simulink model "P2PHVDCMMC"  (R2024a)
settings: Solver=FixedStepDiscrete  StartTime=0.0  StopTime=10  RelTol=1e-3
PreLoadFcn:
  | % HVDCMMCInterconnectionParam
StartFcn:
  | tic
StopFcn:
  | toc
values from neighbouring files (symbols this model uses):
  C_PM = 1.758e-3    (= 0.001758)    [P2PHVDCMMCcode.m]    (also in SFu.mat)
  Cg = 50e-9    (= 5e-08)    [P2PHVDCMMCcode.m]    (also in SFu.mat)
  Fc = Fnom*3.37    (= 168.5)    [P2PHVDCMMCcode.m]    (also in SFu.mat)
  Fnom = 50    [P2PHVDCMMCcode.m]    (also in SFu.mat)
  HRM = 1    [SFu.mat]
  Ki_Ireg = 6    [P2PHVDCMMCcode.m]    (also in SFu.mat)
  Ki_Preg = 1.0    (= 1)    [P2PHVDCMMCcode.m]    (also in SFu.mat)
  Ki_Qreg = 1.0    (= 1)    [P2PHVDCMMCcode.m]    (also in SFu.mat)
  Ki_VDCreg = 100    [P2PHVDCMMCcode.m]    (also in SFu.mat)
  Kp_Ireg = 0.6    [P2PHVDCMMCcode.m]    (also in SFu.mat)
  Kp_Preg = 0.5/3    (= 0.166666666667)    [P2PHVDCMMCcode.m]    (also in SFu.mat)
  Kp_Qreg = 0.5/3    (= 0.166666666667)    [P2PHVDCMMCcode.m]    (also in SFu.mat)
  Kp_VDCreg = 4    [P2PHVDCMMCcode.m]    (also in SFu.mat)
  L_cable = 15e-3    (= 0.015)    [P2PHVDCMMCcode.m]    (also in SFu.mat)
  Larm = Larm_pu*(Zb_ac/(2*pi*Fnom))    [P2PHVDCMMCcode.m]    (also in SFu.mat = 0.0529455974536)
  Larm_pu = 0.15    [P2PHVDCMMCcode.m]    (also in SFu.mat)
  Lff = Larm_pu/2    (= 0.075)    [P2PHVDCMMCcode.m]    (also in SFu.mat)
  Limits_Ireg = [ 2.0  -2.0]    [P2PHVDCMMCcode.m]    (also in SFu.mat = [2 -2])
  Limits_Preg = [ 1.2, 0.8 ]    [P2PHVDCMMCcode.m]    (also in SFu.mat = [1.2 0.8])
  Limits_Qreg = [ 0.25, -0.25 ]    [P2PHVDCMMCcode.m]    (also in SFu.mat = [0.25 -0.25])
  Limits_VDCreg = [ 2.0  -2.0]    [P2PHVDCMMCcode.m]    (also in SFu.mat = [2 -2])
  Lxfo = 0.12    [P2PHVDCMMCcode.m]    (also in SFu.mat)
  N = 1    [P2PHVDCMMCcode.m]    (also in SFu.mat)
  Nb_PM = 36    [P2PHVDCMMCcode.m]    (also in SFu.mat)
  Pnom = 1000e6    (= 1000000000)    [P2PHVDCMMCcode.m]    (also in SFu.mat)
  R_cable = 0.5    [P2PHVDCMMCcode.m]    (also in SFu.mat)
  R_startup = 400    [P2PHVDCMMCcode.m]    (also in SFu.mat)
  Rarm = Rarm_pu*Zb_ac    [P2PHVDCMMCcode.m]    (also in SFu.mat = 0.1663335)
  Rff = Rarm_pu/2    (= 0.00075)    [P2PHVDCMMCcode.m]    (also in SFu.mat)
  Rg = 100    [P2PHVDCMMCcode.m]    (also in SFu.mat)
  Rxfo = 0.003    [P2PHVDCMMCcode.m]    (also in SFu.mat)
  S =     [SFu.mat]
  Slope_Qref = 0.5    [P2PHVDCMMCcode.m]    (also in SFu.mat)
  Slope_Vdc_ref = Vnom_dc/5    (= 128000)    [P2PHVDCMMCcode.m]    (also in SFu.mat)
  Tfault = 9999    [SFu.mat]
  Ts = Ts_Control    (= 4e-05)    [P2PHVDCMMCcode.m]    (also in SFu.mat)
  Ts_Control = 40e-6    (= 4e-05)    [P2PHVDCMMCcode.m]    (also in SFu.mat)
  Ts_dqn = 2e-5    (= 2e-05)    [P2PHVDCMMCcode.m]    (also in SFu.mat)
  Ts_Power = 20e-6    (= 2e-05)    [P2PHVDCMMCcode.m]    (also in SFu.mat)
  Vnom_dc = 640e3    (= 640000)    [P2PHVDCMMCcode.m]    (also in SFu.mat)
  Vnom_prim = 400e3    (= 400000)    [P2PHVDCMMCcode.m]    (also in SFu.mat)
  Vnom_sec = 333e3    (= 333000)    [P2PHVDCMMCcode.m]    (also in SFu.mat)
  Ws = 314.159265359    [SFu.mat]
undefined symbols (not defined in the file or in its folder): DiscIntNeverNeededParam, Discrete, DQN_Lib, gcbh, Int_DQNc_Mat, Mult_DQNc_Mat, Pcc, sps, sps_rtmsupport, spsMeanValueVariableFrequencyModel, spsPLL3phModel, SY3
libraries: simulink x38, spsControlledVoltageSourceLib x30, spsVoltageMeasurementLib x21, spsIdealSwitchLib x21, powerlib_extras x12, spsSecondOrderFilterLib x12, spsCurrentMeasurementLib x12, spsdq0toabcLib x9, spsMeanLib x8, spsMeanVariableFrequencyLib x8, spsabctodq0Lib x8, spsThreePhaseSeriesRLCBranchLib x7
(part 12 of 13)

== matlab function P2PHVDCMMC/Subsystem4/ACinv/Mult_DQNc_Mat3 ==
  data: Xdcpnz_c input; Ydcpnz_c input; N parameter; HrmDbl parameter; Zdcpnz_c output
function Zdcpnz_c    = fMultDQNc(Xdcpnz_c, Ydcpnz_c, N, HrmDbl)
    Zdcpnz_c = complex(zeros(3,2*N+1));

    persistent T132;
    persistent T213;
    persistent T231;
    persistent T321;
    persistent T312;
    persistent Sas;
    persistent Ssa;

    if(isempty(T132)) 
        T132 = [1 0 0; 0 0 1; 0 1 0];
        T213 = [0 1 0; 1 0 0; 0 0 1];
        T231 = [0 1 0; 0 0 1; 1 0 0];
        T321 = [0 0 1; 0 1 0; 1 0 0];
        T312 = [0 0 1; 1 0 0; 0 1 0];

        a = -0.5+0.866i;
        a2 = -0.5-0.866i;
        Sas = [1,a,a2;1,a2,a;1,1,1]/3;
        Ssa = eye(3)/(Sas);
    end

%%%%%%%%%%%%%%%%%%%%%%%%%%%%%%

    Zdcpnz_c(:,1) = Sas*(Ssa*Xdcpnz_c(:,1).*Ssa*Ydcpnz_c(:,1));

    sX = size(Xdcpnz_c,2);
    Xdcpnz_c = [Xdcpnz_c zeros(3,N+1-sX)];

    sY = size(Ydcpnz_c,2);
    Ydcpnz_c = [Ydcpnz_c zeros(3,N+1-sY)];

       
    for h = 1 : 2*N
        if(h<=N)

            Zdcpnz_c(3,1) = Zdcpnz_c(3,1) + 0.5*real(Xdcpnz_c(:,h+1)'*Ydcpnz_c(:,h+1));


            Zdcpnz_c(3,2*h+1) = Zdcpnz_c(3,2*h+1) + 0.5*Xdcpnz_c(1,h+1)*Ydcpnz_c(2,h+1)*exp(-1i*pi/2);

            Zdcpnz_c(1:2,1) = Zdcpnz_c(1:2,1) + 0.25*abs(Xdcpnz_c(1,h+1))*abs(Ydcpnz_c(2,h+1))*[1;1].*exp(1i*((-angle(Xdcpnz_c(1,h+1))+angle(Ydcpnz_c(2,h+1)))*[1;-1]));
            Zdcpnz_c(1:2,1) = Zdcpnz_c(1:2,1) + 0.25*abs(Xdcpnz_c(1,h+1))*abs(Ydcpnz_c(3,h+1))*[1;1].*exp(1i*((-angle(Xdcpnz_c(1,h+1))+angle(Ydcpnz_c(3,h+1)))*[-1;1]));


            Zdcpnz_c(3,2*h+1) = Zdcpnz_c(3,2*h+1) + 0.5*Xdcpnz_c(2,h+1)*Ydcpnz_c(1,h+1)*exp(-1i*pi/2);


            Zdcpnz_c(1:2,1) = Zdcpnz_c(1:2,1) + 0.25*abs(Xdcpnz_c(2,h+1))*abs(Ydcpnz_c(1,h+1))*[1;1].*exp(1i*((-angle(Xdcpnz_c(2,h+1))+angle(Ydcpnz_c(1,h+1)))*[-1;1]));
            Zdcpnz_c(1:2,1) = Zdcpnz_c(1:2,1) + 0.25*abs(Xdcpnz_c(2,h+1))*abs(Ydcpnz_c(3,h+1))*[1;1].*exp(1i*((-angle(Xdcpnz_c(2,h+1))+angle(Ydcpnz_c(3,h+1)))*[1;-1]));
            
            Zdcpnz_c(1:2,1) = Zdcpnz_c(1:2,1) + 0.25*abs(Xdcpnz_c(3,h+1))*abs(Ydcpnz_c(1,h+1))*[1;1].*exp(1i*((-angle(Xdcpnz_c(3,h+1))+angle(Ydcpnz_c(1,h+1)))*[1;-1]));
            Zdcpnz_c(1:2,1) = Zdcpnz_c(1:2,1) + 0.25*abs(Xdcpnz_c(3,h+1))*abs(Ydcpnz_c(2,h+1))*[1;1].*exp(1i*((-angle(Xdcpnz_c(3,h+1))+angle(Ydcpnz_c(2,h+1)))*[-1;+1]));

            %%%%%%%%%%%%%%%%% POSITIVE (Ydc*Xp) %%%%%%%%%%%%%%%%%%%
            Zdcpnz_c(:,h+1) = Zdcpnz_c(:,h+1) + T312*Ydcpnz_c(:,1)*Xdcpnz_c(1,h+1); %[0 0 1; 1 0 0; 0 1 0]
            %%%%%%%%%%%%%%%%% POSITIVE (Xdc*Yp) %%%%%%%%%%%%%%%%%%%
            Zdcpnz_c(:,h+1) = Zdcpnz_c(:,h+1) + T312*Xdcpnz_c(:,1)*Ydcpnz_c(1,h+1);
            %%%%%%%%%%%%%%%%% NEGATIVE (Ydc*Xn) %%%%%%%%%%%%%%%%%%%
            Zdcpnz_c(:,h+1) = Zdcpnz_c(:,h+1) + T231*Ydcpnz_c(:,1)*Xdcpnz_c(2,h+1);
            %%%%%%%%%%%%%%%%% NEGATIVE (Xdc*Yn) %%%%%%%%%%%%%%%%%%%
            Zdcpnz_c(:,h+1) = Zdcpnz_c(:,h+1) + T231*Xdcpnz_c(:,1)*Ydcpnz_c(2,h+1);
            %%%%%%%%%%%%%%%%%%%%%%%%%%%%%%%%%%%%%%%%%%%%%%%%%%%%%%
            Zdcpnz_c(:,h+1) = Zdcpnz_c(:,h+1) + Ydcpnz_c(:,1)*Xdcpnz_c(3,h+1);
            %%%%%%%%%%%%%%%%%%%%%%%%%%%%%%%%%%%%%%%%%%%%%%%%%%%%%%
            Zdcpnz_c(:,h+1) = Zdcpnz_c(:,h+1) + Xdcpnz_c(:,1)*Ydcpnz_c(3,h+1);
            
%%%%%%%%%%%%%%%%%%%%%% h<=N ODD %%%%%%%%%%%%%%%%%%%%%%%%%%%%%%%%%%%%%%%%%
            if(mod(h,2)==1) 
                %%%%%%%%%%%%%%%%% D3p (3ph+) %%%%%%%%%%%%%%%%%%%%%%%

                %&%%%%%%%%%%%%%%%%%%%%%%%%%% PP + NN %%%%%%%%%%%%%%%%%%%%%%%%%%%
                for i = 1 : h - 1
                   Zdcpnz_c(1,h+1) = Zdcpnz_c(1,h+1) +    0.5*( real(Xdcpnz_c(2,i+1))*imag(Ydcpnz_c(2,h-i+1)) + imag(Xdcpnz_c(2,i+1))*real(Ydcpnz_c(2,h-i+1)) );
                   Zdcpnz_c(1,h+1) = Zdcpnz_c(1,h+1) + 1i*0.5*( -real(Xdcpnz_c(2,i+1))*real(Ydcpnz_c(2,h-i+1)) + imag(Xdcpnz_c(2,i+1))*imag(Ydcpnz_c(2,h-i+1)) );

                   Zdcpnz_c(2,h+1) = Zdcpnz_c(2,h+1) +    0.5*( real(Xdcpnz_c(1,i+1))*imag(Ydcpnz_c(1,h-i+1)) + imag(Xdcpnz_c(1,i+1))*real(Ydcpnz_c(1,h-i+1)) );
                   Zdcpnz_c(2,h+1) = Zdcpnz_c(2,h+1) + 1i*0.5*( -real(Xdcpnz_c(1,i+1))*real(Ydcpnz_c(1,h-i+1)) + imag(Xdcpnz_c(1,i+1))*imag(Ydcpnz_c(1,h-i+1)) );
                end

                for i = 1 : N - h

                    Zdcpnz_c(3,h+1) = Zdcpnz_c(3,h+1) -    imag(0.5*Xdcpnz_c(1:2,i+1)'*Ydcpnz_c(1:2,i+h+1)) -    imag(0.5*Ydcpnz_c(1:2,i+1)'*Xdcpnz_c(1:2,i+h+1));
                    Zdcpnz_c(3,h+1) = Zdcpnz_c(3,h+1) + 1i*real(0.5*Xdcpnz_c(1:2,i+1)'*Ydcpnz_c(1:2,i+h+1)) + 1i*real(0.5*Ydcpnz_c(1:2,i+1)'*Xdcpnz_c(1:2,i+h+1));

                end
                %&%%%%%%%%%%%%%%%%%%%%%%%%%% PP + NN %%%%%%%%%%%%%%%%%%%%%%%%%%%

                for k = 1 : (N + mod(N+1,2) - h)/2
                    i = 2*k-1;
                    j = i+h;

                    Zdcpnz_c(1,h+1) = Zdcpnz_c(1,h+1) + (0.5*(Xdcpnz_c(:,i+1)'*T132*T213*Ydcpnz_c(:,j+1))*exp(+1i*pi/2)) ...
                                                      + (0.5*(Xdcpnz_c(:,j+1)'*T213*T132*Ydcpnz_c(:,i+1))*exp(-1i*pi/2))';

                    Zdcpnz_c(2,h+1) = Zdcpnz_c(2,h+1) + (0.5*(Xdcpnz_c(:,i+1)'*T132*T321*Ydcpnz_c(:,j+1))*exp(+1i*pi/2)) ...
                                                      + (0.5*(Xdcpnz_c(:,j+1)'*T321*T132*Ydcpnz_c(:,i+1))*exp(-1i*pi/2))';

                    Zdcpnz_c(3,h+1) = Zdcpnz_c(3,h+1) + (0.5*Xdcpnz_c(3,i+1)'*Ydcpnz_c(3,j+1)*exp(1i*pi/2)) ...
                                                      - (0.5*Xdcpnz_c(3,j+1)'*Ydcpnz_c(3,i+1)*exp(1i*pi/2))';
                end

                for k = 1 : (N + mod(N,2) - h - 1)/2
                    i = 2*k;
                    j = i+h;
                    
                    Zdcpnz_c(1,h+1) = Zdcpnz_c(1,h+1) + (0.5*(Xdcpnz_c(:,i+1)'*T132*T213*Ydcpnz_c(:,j+1))*exp(+1i*pi/2)) ...
                                                      + (0.5*(Xdcpnz_c(:,j+1)'*T213*T132*Ydcpnz_c(:,i+1))*exp(-1i*pi/2))';

                    Zdcpnz_c(2,h+1) = Zdcpnz_c(2,h+1) + (0.5*(Xdcpnz_c(:,i+1)'*T132*T321*Ydcpnz_c(:,j+1))*exp(+1i*pi/2)) ...
                                                      + (0.5*(Xdcpnz_c(:,j+1)'*T321*T132*Ydcpnz_c(:,i+1))*exp(-1i*pi/2))';

                    Zdcpnz_c(3,h+1) = Zdcpnz_c(3,h+1) + (0.5*Xdcpnz_c(3,i+1)'*Ydcpnz_c(3,j+1)*exp(1i*pi/2)) ...
                                                      - (0.5*Xdcpnz_c(3,j+1)'*Ydcpnz_c(3,i+1)*exp(1i*pi/2))';
                end

                for k = (h-1)/2:-1:1
                    i = k;
                    j = h-i;  

                    Zdcpnz_c(3,h+1) = Zdcpnz_c(3,h+1) + 0.5*(real(Xdcpnz_c(:,i+1))'*T213*imag(Ydcpnz_c(:,j+1)) + imag(Xdcpnz_c(:,i+1))'*T213*real(Ydcpnz_c(:,j+1)) ...
                                                           + real(Xdcpnz_c(:,j+1))'*T213*imag(Ydcpnz_c(:,i+1)) + imag(Xdcpnz_c(:,j+1))'*T213*real(Ydcpnz_c(:,i+1)));
                                                                                       
                    Zdcpnz_c(3,h+1) = Zdcpnz_c(3,h+1) + 1i*0.5*(-real(Xdcpnz_c(:,i+1))'*T213*real(Ydcpnz_c(:,j+1)) + imag(Xdcpnz_c(:,i+1))'*T213*imag(Ydcpnz_c(:,j+1)) ...
                                                           - real(Xdcpnz_c(:,j+1))'*T213*real(Ydcpnz_c(:,i+1)) + imag(Xdcpnz_c(:,j+1))'*T213*imag(Ydcpnz_c(:,i+1)));

                    Zdcpnz_c(1,h+1) = Zdcpnz_c(1,h+1) + 0.5*(real(Xdcpnz_c([1,3],i+1))'*[0 1; 1 0]*imag(Ydcpnz_c([1,3],j+1)) + imag(Xdcpnz_c([1,3],i+1))'*[0 1; 1 0]*real(Ydcpnz_c([1,3],j+1)) ...
                                                           + real(Xdcpnz_c([1,3],j+1))'*[0 1; 1 0]*imag(Ydcpnz_c([1,3],i+1)) + imag(Xdcpnz_c([1,3],j+1))'*[0 1; 1 0]*real(Ydcpnz_c([1,3],i+1)) );

                    Zdcpnz_c(1,h+1) = Zdcpnz_c(1,h+1) + 1i*0.5*(-real(Xdcpnz_c([1,3],i+1))'*[0 1; 1 0]*real(Ydcpnz_c([1,3],j+1)) + imag(Xdcpnz_c([1,3],i+1))'*[0 1; 1 0]*imag(Ydcpnz_c([1,3],j+1)) ...
                                                              - real(Xdcpnz_c([1,3],j+1))'*[0 1; 1 0]*real(Ydcpnz_c([1,3],i+1)) + imag(Xdcpnz_c([1,3],j+1))'*[0 1; 1 0]*imag(Ydcpnz_c([1,3],i+1)) );

                    Zdcpnz_c(2,h+1) = Zdcpnz_c(2,h+1) + 0.5*(real(Xdcpnz_c([2,3],i+1))'*[0 1; 1 0]*imag(Ydcpnz_c([2,3],j+1)) + imag(Xdcpnz_c([2,3],i+1))'*[0 1; 1 0]*real(Ydcpnz_c([2,3],j+1)) ...
                                                           + real(Xdcpnz_c([2,3],j+1))'*[0 1; 1 0]*imag(Ydcpnz_c([2,3],i+1)) + imag(Xdcpnz_c([2,3],j+1))'*[0 1; 1 0]*real(Ydcpnz_c([2,3],i+1)) );

                    Zdcpnz_c(2,h+1) = Zdcpnz_c(2,h+1) + 1i*0.5*(-real(Xdcpnz_c([2,3],i+1))'*[0 1; 1 0]*real(Ydcpnz_c([2,3],j+1)) + imag(Xdcpnz_c([2,3],i+1))'*[0 1; 1 0]*imag(Ydcpnz_c([2,3],j+1)) ...
                                                              - real(Xdcpnz_c([2,3],j+1))'*[0 1; 1 0]*real(Ydcpnz_c([2,3],i+1)) + imag(Xdcpnz_c([2,3],j+1))'*[0 1; 1 0]*imag(Ydcpnz_c([2,3],i+1)) );

                end
%%%%%%%%%%%%%%%%%%%%%% h<=N EVEN %%%%%%%%%%%%%%%%%%%%%%%%%%%%%%%%%%%%%%%%%           
            else  

                Zdcpnz_c(3,h+1) = Zdcpnz_c(3,h+1) + 0.5*imag(Xdcpnz_c(3,h/2+1)*Ydcpnz_c(3,h/2+1))           -0.5*1i*real(Xdcpnz_c(3,h/2+1)*Ydcpnz_c(3,h/2+1));
                Zdcpnz_c(1,h+1) = Zdcpnz_c(1,h+1) + 0.5*real(Xdcpnz_c(:,h/2+1))'*T321*imag(Ydcpnz_c(:,h/2+1)) + 0.5*imag(Xdcpnz_c(:,h/2+1))'*T321*real(Ydcpnz_c(:,h/2+1));
                Zdcpnz_c(1,h+1) = Zdcpnz_c(1,h+1) - 0.5*1i*real(Xdcpnz_c(:,h/2+1))'*T321*real(Ydcpnz_c(:,h/2+1)) + 0.5*1i*imag(Xdcpnz_c(:,h/2+1))'*T321*imag(Ydcpnz_c(:,h/2+1));
                Zdcpnz_c(2,h+1) = Zdcpnz_c(2,h+1) + 0.5*real(Xdcpnz_c(:,h/2+1))'*T132*imag(Ydcpnz_c(:,h/2+1)) + 0.5*imag(Xdcpnz_c(:,h/2+1))'*T132*real(Ydcpnz_c(:,h/2+1));
                Zdcpnz_c(2,h+1) = Zdcpnz_c(2,h+1) - 0.5*1i*real(Xdcpnz_c(:,h/2+1))'*T132*real(Ydcpnz_c(:,h/2+1)) + 0.5*1i*imag(Xdcpnz_c(:,h/2+1))'*T132*imag(Ydcpnz_c(:,h/2+1));
                
                for k = 1:N-h
                    i = k;
                    j = h+i;

                    Zdcpnz_c(1,h+1) = Zdcpnz_c(1,h+1) + 0.5*( - real(Xdcpnz_c(:,i+1))'*T231*imag(Ydcpnz_c(:,j+1)) + imag(Xdcpnz_c(:,i+1))'*T231*real(Ydcpnz_c(:,j+1)) ...
                                                              + real(Xdcpnz_c(:,j+1))'*T312*imag(Ydcpnz_c(:,i+1)) - imag(Xdcpnz_c(:,j+1))'*T312*real(Ydcpnz_c(:,i+1)));

                    Zdcpnz_c(1,h+1) = Zdcpnz_c(1,h+1) + 0.5*1i*( + real(Xdcpnz_c(:,i+1))'*T231*real(Ydcpnz_c(:,j+1)) + imag(Xdcpnz_c(:,i+1))'*T231*imag(Ydcpnz_c(:,j+1)) ...
                                                                 + real(Xdcpnz_c(:,j+1))'*T312*real(Ydcpnz_c(:,i+1)) + imag(Xdcpnz_c(:,j+1))'*T312*imag(Ydcpnz_c(:,i+1)));

                    Zdcpnz_c(2,h+1) = Zdcpnz_c(2,h+1) + 0.5*( - real(Xdcpnz_c(:,i+1))'*T312*imag(Ydcpnz_c(:,j+1)) + imag(Xdcpnz_c(:,i+1))'*T312*real(Ydcpnz_c(:,j+1)) ...
                                                              + real(Xdcpnz_c(:,j+1))'*T231*imag(Ydcpnz_c(:,i+1)) - imag(Xdcpnz_c(:,j+1))'*T231*real(Ydcpnz_c(:,i+1)));

                    Zdcpnz_c(2,h+1) = Zdcpnz_c(2,h+1) + 1i*0.5*( + real(Xdcpnz_c(:,i+1))'*T312*real(Ydcpnz_c(:,j+1)) + imag(Xdcpnz_c(:,i+1))'*T312*imag(Ydcpnz_c(:,j+1)) ...
                                                              + real(Xdcpnz_c(:,j+1))'*T231*real(Ydcpnz_c(:,i+1)) + imag(Xdcpnz_c(:,j+1))'*T231*imag(Ydcpnz_c(:,i+1)));

                    Zdcpnz_c(3,h+1) = Zdcpnz_c(3,h+1) + 0.5*(-real(Xdcpnz_c(:,i+1))'*imag(Ydcpnz_c(:,j+1))+imag(Xdcpnz_c(:,i+1))'*real(Ydcpnz_c(:,j+1)) ...
                                                             +real(Xdcpnz_c(:,j+1))'*imag(Ydcpnz_c(:,i+1))-imag(Xdcpnz_c(:,j+1))'*real(Ydcpnz_c(:,i+1)));

                    Zdcpnz_c(3,h+1) = Zdcpnz_c(3,h+1) + 0.5*1i*(+real(Xdcpnz_c(:,i+1))'*real(Ydcpnz_c(:,j+1))+imag(Xdcpnz_c(:,i+1))'*imag(Ydcpnz_c(:,j+1)) ...
                                                             +real(Xdcpnz_c(:,j+1))'*real(Ydcpnz_c(:,i+1))+imag(Xdcpnz_c(:,j+1))'*imag(Ydcpnz_c(:,i+1)));

                end

                for k = h/2-1:-1:1
                    i = k;
                    j = h-i;   

                    Zdcpnz_c(3,h+1) = Zdcpnz_c(3,h+1) +    0.5*(+real(Xdcpnz_c(:,i+1))'*T213*imag(Ydcpnz_c(:,j+1)) + real(Xdcpnz_c(:,j+1))'*T213*imag(Ydcpnz_c(:,i+1)) + imag(Xdcpnz_c(:,i+1))'*T213*real(Ydcpnz_c(:,j+1)) + imag(Xdcpnz_c(:,j+1))'*T213*real(Ydcpnz_c(:,i+1)));

                    Zdcpnz_c(3,h+1) = Zdcpnz_c(3,h+1) + 1i*0.5*(-real(Xdcpnz_c(:,i+1))'*T213*real(Ydcpnz_c(:,j+1)) - real(Xdcpnz_c(:,j+1))'*T213*real(Ydcpnz_c(:,i+1)) + imag(Xdcpnz_c(:,i+1))'*T213*imag(Ydcpnz_c(:,j+1)) + imag(Xdcpnz_c(:,j+1))'*T213*imag(Ydcpnz_c(:,i+1)));

                    Zdcpnz_c(1,h+1) = Zdcpnz_c(1,h+1) + 0.5*( + real(Xdcpnz_c(:,i+1))'*T321*imag(Ydcpnz_c(:,j+1)) + imag(Xdcpnz_c(:,i+1))'*T321*real(Ydcpnz_c(:,j+1)) ...
                                                              + real(Xdcpnz_c(:,j+1))'*T321*imag(Ydcpnz_c(:,i+1)) + imag(Xdcpnz_c(:,j+1))'*T321*real(Ydcpnz_c(:,i+1)));


                    Zdcpnz_c(1,h+1) = Zdcpnz_c(1,h+1) + 0.5*1i*( - real(Xdcpnz_c(:,i+1))'*T321*real(Ydcpnz_c(:,j+1)) + imag(Xdcpnz_c(:,i+1))'*T321*imag(Ydcpnz_c(:,j+1)) ...
                                                                 - real(Xdcpnz_c(:,j+1))'*T321*real(Ydcpnz_c(:,i+1)) + imag(Xdcpnz_c(:,j+1))'*T321*imag(Ydcpnz_c(:,i+1)));
                    
                    Zdcpnz_c(2,h+1) = Zdcpnz_c(2,h+1) + 0.5*( + real(Xdcpnz_c(:,i+1))'*T132*imag(Ydcpnz_c(:,j+1)) + imag(Xdcpnz_c(:,i+1))'*T132*real(Ydcpnz_c(:,j+1)) ...
                                                              + real(Xdcpnz_c(:,j+1))'*T132*imag(Ydcpnz_c(:,i+1)) + imag(Xdcpnz_c(:,j+1))'*T132*real(Ydcpnz_c(:,i+1)));

                    Zdcpnz_c(2,h+1) = Zdcpnz_c(2,h+1) + 1i*0.5*( - real(Xdcpnz_c(:,i+1))'*T132*real(Ydcpnz_c(:,j+1)) + imag(Xdcpnz_c(:,i+1))'*T132*imag(Ydcpnz_c(:,j+1)) ...
                                                                 - real(Xdcpnz_c(:,j+1))'*T132*real(Ydcpnz_c(:,i+1)) + imag(Xdcpnz_c(:,j+1))'*T132*imag(Ydcpnz_c(:,i+1)));

                end
            end
%%%%%%%%%%%%%%%%%%%%%%%%%%%% h>N  %%%%%%%%%%%%%%%%%%%%%%%%%%%%%%%%%%%%%%%%% 
        else %h>N
            if(HrmDbl)
            
                %%%%%%%%%%%%%%%%%%%%%%%%%%% PP + NN %%%%%%%%%%%%%%%%%%%%%%%%%%%
                for i = h-N : N
                    Zdcpnz_c(1,h+1) = Zdcpnz_c(1,h+1) +    0.5*( real(Xdcpnz_c(2,i+1))*imag(Ydcpnz_c(2,h-i+1)) + imag(Xdcpnz_c(2,i+1))*real(Ydcpnz_c(2,h-i+1)) );
                    Zdcpnz_c(1,h+1) = Zdcpnz_c(1,h+1) + 1i*0.5*( -real(Xdcpnz_c(2,i+1))*real(Ydcpnz_c(2,h-i+1)) + imag(Xdcpnz_c(2,i+1))*imag(Ydcpnz_c(2,h-i+1)) );

                    Zdcpnz_c(2,h+1) = Zdcpnz_c(2,h+1) +    0.5*( real(Xdcpnz_c(1,i+1))*imag(Ydcpnz_c(1,h-i+1)) + imag(Xdcpnz_c(1,i+1))*real(Ydcpnz_c(1,h-i+1)) );
                    Zdcpnz_c(2,h+1) = Zdcpnz_c(2,h+1) + 1i*0.5*( -real(Xdcpnz_c(1,i+1))*real(Ydcpnz_c(1,h-i+1)) + imag(Xdcpnz_c(1,i+1))*imag(Ydcpnz_c(1,h-i+1)) );
                end
                %%%%%%%%%%%%%%%%%%%%%%%%%%% PP + NN %%%%%%%%%%%%%%%%%%%%%%%%%%%

                if(mod(h,2)==1) %%%%%%%%%%% h>N ODD %%%%%%%%%%%%%%%%%%%

                    for k = (h-1)/2:-1:h-N
                        i = k;  %%%
                        j = h-i;

                        Zdcpnz_c(1,h+1) = Zdcpnz_c(1,h+1) + 0.5*( + real(Xdcpnz_c([1,3],i+1))'*imag(Ydcpnz_c([3,1],j+1)) + imag(Xdcpnz_c([1,3],i+1))'*real(Ydcpnz_c([3,1],j+1)) ...
                                                                  + real(Xdcpnz_c([1,3],j+1))'*imag(Ydcpnz_c([3,1],i+1)) + imag(Xdcpnz_c([1,3],j+1))'*real(Ydcpnz_c([3,1],i+1)));

                        Zdcpnz_c(1,h+1) = Zdcpnz_c(1,h+1) + 1i*0.5*( - real(Xdcpnz_c([1,3],i+1))'*real(Ydcpnz_c([3,1],j+1)) + imag(Xdcpnz_c([1,3],i+1))'*imag(Ydcpnz_c([3,1],j+1)) ...
                                                                     - real(Xdcpnz_c([1,3],j+1))'*real(Ydcpnz_c([3,1],i+1)) + imag(Xdcpnz_c([1,3],j+1))'*imag(Ydcpnz_c([3,1],i+1)));

                        Zdcpnz_c(2,h+1) = Zdcpnz_c(2,h+1) + 0.5*( + real(Xdcpnz_c([2,3],i+1))'*imag(Ydcpnz_c([3,2],j+1)) + imag(Xdcpnz_c([2,3],i+1))'*real(Ydcpnz_c([3,2],j+1)) ...
                                                                  + real(Xdcpnz_c([2,3],j+1))'*imag(Ydcpnz_c([3,2],i+1)) + imag(Xdcpnz_c([2,3],j+1))'*real(Ydcpnz_c([3,2],i+1)));

                        Zdcpnz_c(2,h+1) = Zdcpnz_c(2,h+1) + 1i*0.5*( - real(Xdcpnz_c([2,3],i+1))'*real(Ydcpnz_c([3,2],j+1)) + imag(Xdcpnz_c([2,3],i+1))'*imag(Ydcpnz_c([3,2],j+1)) ...
                                                                     - real(Xdcpnz_c([2,3],j+1))'*real(Ydcpnz_c([3,2],i+1)) + imag(Xdcpnz_c([2,3],j+1))'*imag(Ydcpnz_c([3,2],i+1)));

                        Zdcpnz_c(3,h+1) = Zdcpnz_c(3,h+1) +    0.5*(+real(Xdcpnz_c(:,i+1))'*T213*imag(Ydcpnz_c(:,j+1)) + real(Xdcpnz_c(:,j+1))'*T213*imag(Ydcpnz_c(:,i+1)) + imag(Xdcpnz_c(:,i+1))'*T213*real(Ydcpnz_c(:,j+1)) + imag(Xdcpnz_c(:,j+1))'*T213*real(Ydcpnz_c(:,i+1)));
                        Zdcpnz_c(3,h+1) = Zdcpnz_c(3,h+1) + 1i*0.5*(-real(Xdcpnz_c(:,i+1))'*T213*real(Ydcpnz_c(:,j+1)) - real(Xdcpnz_c(:,j+1))'*T213*real(Ydcpnz_c(:,i+1)) + imag(Xdcpnz_c(:,i+1))'*T213*imag(Ydcpnz_c(:,j+1)) + imag(Xdcpnz_c(:,j+1))'*T213*imag(Ydcpnz_c(:,i+1)));

                    end

                else %%%%%%%%%%% h>N EVEN %%%%%%%%%%%%%%%%%%%

                    Zdcpnz_c(1,h+1) = 0.5*real(Xdcpnz_c(:,h/2+1))'*T321*imag(Ydcpnz_c(:,h/2+1)) + 0.5*imag(Xdcpnz_c(:,h/2+1))'*T321*real(Ydcpnz_c(:,h/2+1)) - 0.5*1i*real(Xdcpnz_c(:,h/2+1))'*T321*real(Ydcpnz_c(:,h/2+1)) + 0.5*1i*imag(Xdcpnz_c(:,h/2+1))'*T321*imag(Ydcpnz_c(:,h/2+1));
                    Zdcpnz_c(2,h+1) = 0.5*real(Xdcpnz_c(:,h/2+1))'*T132*imag(Ydcpnz_c(:,h/2+1)) + 0.5*imag(Xdcpnz_c(:,h/2+1))'*T132*real(Ydcpnz_c(:,h/2+1))- 0.5*1i*real(Xdcpnz_c(:,h/2+1))'*T132*real(Ydcpnz_c(:,h/2+1)) + 0.5*1i*imag(Xdcpnz_c(:,h/2+1))'*T132*imag(Ydcpnz_c(:,h/2+1));
                    Zdcpnz_c(3,h+1) = Zdcpnz_c(3,h+1) + 0.5*imag(Xdcpnz_c(3,h/2+1)*Ydcpnz_c(3,h/2+1)) - 1i*0.5*real(Xdcpnz_c(3,h/2+1)*Ydcpnz_c(3,h/2+1));


                    for i = (h+2)/2:N
                        j = h-i;

                        Zdcpnz_c(1,h+1) = Zdcpnz_c(1,h+1) + 0.5*( + real(Xdcpnz_c(:,i+1))'*T321*imag(Ydcpnz_c(:,j+1)) + imag(Xdcpnz_c(:,i+1))'*T321*real(Ydcpnz_c(:,j+1)) ...
                                                                  + real(Xdcpnz_c(:,j+1))'*T321*imag(Ydcpnz_c(:,i+1)) + imag(Xdcpnz_c(:,j+1))'*T321*real(Ydcpnz_c(:,i+1)));
    
                        Zdcpnz_c(1,h+1) = Zdcpnz_c(1,h+1) + 0.5*1i*( - real(Xdcpnz_c(:,i+1))'*T321*real(Ydcpnz_c(:,j+1)) + imag(Xdcpnz_c(:,i+1))'*T321*imag(Ydcpnz_c(:,j+1)) ...
                                                                     - real(Xdcpnz_c(:,j+1))'*T321*real(Ydcpnz_c(:,i+1)) + imag(Xdcpnz_c(:,j+1))'*T321*imag(Ydcpnz_c(:,i+1)));

                        Zdcpnz_c(2,h+1) = Zdcpnz_c(2,h+1) + 0.5*( + real(Xdcpnz_c(:,i+1))'*T132*imag(Ydcpnz_c(:,j+1)) + imag(Xdcpnz_c(:,i+1))'*T132*real(Ydcpnz_c(:,j+1)) ...
                                                                  + real(Xdcpnz_c(:,j+1))'*T132*imag(Ydcpnz_c(:,i+1)) + imag(Xdcpnz_c(:,j+1))'*T132*real(Ydcpnz_c(:,i+1)));
    
                        Zdcpnz_c(2,h+1) = Zdcpnz_c(2,h+1) + 0.5*1i*( - real(Xdcpnz_c(:,i+1))'*T132*real(Ydcpnz_c(:,j+1)) + imag(Xdcpnz_c(:,i+1))'*T132*imag(Ydcpnz_c(:,j+1)) ...
                                                                     - real(Xdcpnz_c(:,j+1))'*T132*real(Ydcpnz_c(:,i+1)) + imag(Xdcpnz_c(:,j+1))'*T132*imag(Ydcpnz_c(:,i+1)));

                        Zdcpnz_c(3,h+1) = Zdcpnz_c(3,h+1) +    0.5*(+real(Xdcpnz_c(:,i+1))'*T213*imag(Ydcpnz_c(:,j+1)) + real(Xdcpnz_c(:,j+1))'*T213*imag(Ydcpnz_c(:,i+1)) + imag(Xdcpnz_c(:,i+1))'*T213*real(Ydcpnz_c(:,j+1)) + imag(Xdcpnz_c(:,j+1))'*T213*real(Ydcpnz_c(:,i+1)));
                        Zdcpnz_c(3,h+1) = Zdcpnz_c(3,h+1) + 1i*0.5*(-real(Xdcpnz_c(:,i+1))'*T213*real(Ydcpnz_c(:,j+1)) - real(Xdcpnz_c(:,j+1))'*T213*real(Ydcpnz_c(:,i+1)) + imag(Xdcpnz_c(:,i+1))'*T213*imag(Ydcpnz_c(:,j+1)) + imag(Xdcpnz_c(:,j+1))'*T213*imag(Ydcpnz_c(:,i+1)));

                    end
                end
            end
        end  
    end
    

end

== matlab function P2PHVDCMMC/Subsystem4/ACinv/Mult_DQNc_Mat4 ==
  data: Xdcpnz_c input; Ydcpnz_c input; N parameter; HrmDbl parameter; Zdcpnz_c output
function Zdcpnz_c    = fMultDQNc(Xdcpnz_c, Ydcpnz_c, N, HrmDbl)
    Zdcpnz_c = complex(zeros(3,2*N+1));

    persistent T132;
    persistent T213;
    persistent T231;
    persistent T321;
    persistent T312;
    persistent Sas;
    persistent Ssa;

    if(isempty(T132)) 
        T132 = [1 0 0; 0 0 1; 0 1 0];
        T213 = [0 1 0; 1 0 0; 0 0 1];
        T231 = [0 1 0; 0 0 1; 1 0 0];
        T321 = [0 0 1; 0 1 0; 1 0 0];
        T312 = [0 0 1; 1 0 0; 0 1 0];

        a = -0.5+0.866i;
        a2 = -0.5-0.866i;
        Sas = [1,a,a2;1,a2,a;1,1,1]/3;
        Ssa = eye(3)/(Sas);
    end

%%%%%%%%%%%%%%%%%%%%%%%%%%%%%%

    Zdcpnz_c(:,1) = Sas*(Ssa*Xdcpnz_c(:,1).*Ssa*Ydcpnz_c(:,1));

    sX = size(Xdcpnz_c,2);
    Xdcpnz_c = [Xdcpnz_c zeros(3,N+1-sX)];

    sY = size(Ydcpnz_c,2);
    Ydcpnz_c = [Ydcpnz_c zeros(3,N+1-sY)];

       
    for h = 1 : 2*N
        if(h<=N)

            Zdcpnz_c(3,1) = Zdcpnz_c(3,1) + 0.5*real(Xdcpnz_c(:,h+1)'*Ydcpnz_c(:,h+1));


            Zdcpnz_c(3,2*h+1) = Zdcpnz_c(3,2*h+1) + 0.5*Xdcpnz_c(1,h+1)*Ydcpnz_c(2,h+1)*exp(-1i*pi/2);

            Zdcpnz_c(1:2,1) = Zdcpnz_c(1:2,1) + 0.25*abs(Xdcpnz_c(1,h+1))*abs(Ydcpnz_c(2,h+1))*[1;1].*exp(1i*((-angle(Xdcpnz_c(1,h+1))+angle(Ydcpnz_c(2,h+1)))*[1;-1]));
            Zdcpnz_c(1:2,1) = Zdcpnz_c(1:2,1) + 0.25*abs(Xdcpnz_c(1,h+1))*abs(Ydcpnz_c(3,h+1))*[1;1].*exp(1i*((-angle(Xdcpnz_c(1,h+1))+angle(Ydcpnz_c(3,h+1)))*[-1;1]));


            Zdcpnz_c(3,2*h+1) = Zdcpnz_c(3,2*h+1) + 0.5*Xdcpnz_c(2,h+1)*Ydcpnz_c(1,h+1)*exp(-1i*pi/2);


            Zdcpnz_c(1:2,1) = Zdcpnz_c(1:2,1) + 0.25*abs(Xdcpnz_c(2,h+1))*abs(Ydcpnz_c(1,h+1))*[1;1].*exp(1i*((-angle(Xdcpnz_c(2,h+1))+angle(Ydcpnz_c(1,h+1)))*[-1;1]));
            Zdcpnz_c(1:2,1) = Zdcpnz_c(1:2,1) + 0.25*abs(Xdcpnz_c(2,h+1))*abs(Ydcpnz_c(3,h+1))*[1;1].*exp(1i*((-angle(Xdcpnz_c(2,h+1))+angle(Ydcpnz_c(3,h+1)))*[1;-1]));
            
            Zdcpnz_c(1:2,1) = Zdcpnz_c(1:2,1) + 0.25*abs(Xdcpnz_c(3,h+1))*abs(Ydcpnz_c(1,h+1))*[1;1].*exp(1i*((-angle(Xdcpnz_c(3,h+1))+angle(Ydcpnz_c(1,h+1)))*[1;-1]));
            Zdcpnz_c(1:2,1) = Zdcpnz_c(1:2,1) + 0.25*abs(Xdcpnz_c(3,h+1))*abs(Ydcpnz_c(2,h+1))*[1;1].*exp(1i*((-angle(Xdcpnz_c(3,h+1))+angle(Ydcpnz_c(2,h+1)))*[-1;+1]));

            %%%%%%%%%%%%%%%%% POSITIVE (Ydc*Xp) %%%%%%%%%%%%%%%%%%%
            Zdcpnz_c(:,h+1) = Zdcpnz_c(:,h+1) + T312*Ydcpnz_c(:,1)*Xdcpnz_c(1,h+1); %[0 0 1; 1 0 0; 0 1 0]
            %%%%%%%%%%%%%%%%% POSITIVE (Xdc*Yp) %%%%%%%%%%%%%%%%%%%
            Zdcpnz_c(:,h+1) = Zdcpnz_c(:,h+1) + T312*Xdcpnz_c(:,1)*Ydcpnz_c(1,h+1);
            %%%%%%%%%%%%%%%%% NEGATIVE (Ydc*Xn) %%%%%%%%%%%%%%%%%%%
            Zdcpnz_c(:,h+1) = Zdcpnz_c(:,h+1) + T231*Ydcpnz_c(:,1)*Xdcpnz_c(2,h+1);
            %%%%%%%%%%%%%%%%% NEGATIVE (Xdc*Yn) %%%%%%%%%%%%%%%%%%%
            Zdcpnz_c(:,h+1) = Zdcpnz_c(:,h+1) + T231*Xdcpnz_c(:,1)*Ydcpnz_c(2,h+1);
            %%%%%%%%%%%%%%%%%%%%%%%%%%%%%%%%%%%%%%%%%%%%%%%%%%%%%%
            Zdcpnz_c(:,h+1) = Zdcpnz_c(:,h+1) + Ydcpnz_c(:,1)*Xdcpnz_c(3,h+1);
            %%%%%%%%%%%%%%%%%%%%%%%%%%%%%%%%%%%%%%%%%%%%%%%%%%%%%%
            Zdcpnz_c(:,h+1) = Zdcpnz_c(:,h+1) + Xdcpnz_c(:,1)*Ydcpnz_c(3,h+1);
            
%%%%%%%%%%%%%%%%%%%%%% h<=N ODD %%%%%%%%%%%%%%%%%%%%%%%%%%%%%%%%%%%%%%%%%
            if(mod(h,2)==1) 
                %%%%%%%%%%%%%%%%% D3p (3ph+) %%%%%%%%%%%%%%%%%%%%%%%

                %&%%%%%%%%%%%%%%%%%%%%%%%%%% PP + NN %%%%%%%%%%%%%%%%%%%%%%%%%%%
                for i = 1 : h - 1
                   Zdcpnz_c(1,h+1) = Zdcpnz_c(1,h+1) +    0.5*( real(Xdcpnz_c(2,i+1))*imag(Ydcpnz_c(2,h-i+1)) + imag(Xdcpnz_c(2,i+1))*real(Ydcpnz_c(2,h-i+1)) );
                   Zdcpnz_c(1,h+1) = Zdcpnz_c(1,h+1) + 1i*0.5*( -real(Xdcpnz_c(2,i+1))*real(Ydcpnz_c(2,h-i+1)) + imag(Xdcpnz_c(2,i+1))*imag(Ydcpnz_c(2,h-i+1)) );

                   Zdcpnz_c(2,h+1) = Zdcpnz_c(2,h+1) +    0.5*( real(Xdcpnz_c(1,i+1))*imag(Ydcpnz_c(1,h-i+1)) + imag(Xdcpnz_c(1,i+1))*real(Ydcpnz_c(1,h-i+1)) );
                   Zdcpnz_c(2,h+1) = Zdcpnz_c(2,h+1) + 1i*0.5*( -real(Xdcpnz_c(1,i+1))*real(Ydcpnz_c(1,h-i+1)) + imag(Xdcpnz_c(1,i+1))*imag(Ydcpnz_c(1,h-i+1)) );
                end

                for i = 1 : N - h

                    Zdcpnz_c(3,h+1) = Zdcpnz_c(3,h+1) -    imag(0.5*Xdcpnz_c(1:2,i+1)'*Ydcpnz_c(1:2,i+h+1)) -    imag(0.5*Ydcpnz_c(1:2,i+1)'*Xdcpnz_c(1:2,i+h+1));
                    Zdcpnz_c(3,h+1) = Zdcpnz_c(3,h+1) + 1i*real(0.5*Xdcpnz_c(1:2,i+1)'*Ydcpnz_c(1:2,i+h+1)) + 1i*real(0.5*Ydcpnz_c(1:2,i+1)'*Xdcpnz_c(1:2,i+h+1));

                end
                %&%%%%%%%%%%%%%%%%%%%%%%%%%% PP + NN %%%%%%%%%%%%%%%%%%%%%%%%%%%

                for k = 1 : (N + mod(N+1,2) - h)/2
                    i = 2*k-1;
                    j = i+h;

                    Zdcpnz_c(1,h+1) = Zdcpnz_c(1,h+1) + (0.5*(Xdcpnz_c(:,i+1)'*T132*T213*Ydcpnz_c(:,j+1))*exp(+1i*pi/2)) ...
                                                      + (0.5*(Xdcpnz_c(:,j+1)'*T213*T132*Ydcpnz_c(:,i+1))*exp(-1i*pi/2))';

                    Zdcpnz_c(2,h+1) = Zdcpnz_c(2,h+1) + (0.5*(Xdcpnz_c(:,i+1)'*T132*T321*Ydcpnz_c(:,j+1))*exp(+1i*pi/2)) ...
                                                      + (0.5*(Xdcpnz_c(:,j+1)'*T321*T132*Ydcpnz_c(:,i+1))*exp(-1i*pi/2))';

                    Zdcpnz_c(3,h+1) = Zdcpnz_c(3,h+1) + (0.5*Xdcpnz_c(3,i+1)'*Ydcpnz_c(3,j+1)*exp(1i*pi/2)) ...
                                                      - (0.5*Xdcpnz_c(3,j+1)'*Ydcpnz_c(3,i+1)*exp(1i*pi/2))';
                end

                for k = 1 : (N + mod(N,2) - h - 1)/2
                    i = 2*k;
                    j = i+h;
                    
                    Zdcpnz_c(1,h+1) = Zdcpnz_c(1,h+1) + (0.5*(Xdcpnz_c(:,i+1)'*T132*T213*Ydcpnz_c(:,j+1))*exp(+1i*pi/2)) ...
                                                      + (0.5*(Xdcpnz_c(:,j+1)'*T213*T132*Ydcpnz_c(:,i+1))*exp(-1i*pi/2))';

                    Zdcpnz_c(2,h+1) = Zdcpnz_c(2,h+1) + (0.5*(Xdcpnz_c(:,i+1)'*T132*T321*Ydcpnz_c(:,j+1))*exp(+1i*pi/2)) ...
                                                      + (0.5*(Xdcpnz_c(:,j+1)'*T321*T132*Ydcpnz_c(:,i+1))*exp(-1i*pi/2))';

                    Zdcpnz_c(3,h+1) = Zdcpnz_c(3,h+1) + (0.5*Xdcpnz_c(3,i+1)'*Ydcpnz_c(3,j+1)*exp(1i*pi/2)) ...
                                                      - (0.5*Xdcpnz_c(3,j+1)'*Ydcpnz_c(3,i+1)*exp(1i*pi/2))';
                end

                for k = (h-1)/2:-1:1
                    i = k;
                    j = h-i;  

                    Zdcpnz_c(3,h+1) = Zdcpnz_c(3,h+1) + 0.5*(real(Xdcpnz_c(:,i+1))'*T213*imag(Ydcpnz_c(:,j+1)) + imag(Xdcpnz_c(:,i+1))'*T213*real(Ydcpnz_c(:,j+1)) ...
                                                           + real(Xdcpnz_c(:,j+1))'*T213*imag(Ydcpnz_c(:,i+1)) + imag(Xdcpnz_c(:,j+1))'*T213*real(Ydcpnz_c(:,i+1)));
                                                                                       
                    Zdcpnz_c(3,h+1) = Zdcpnz_c(3,h+1) + 1i*0.5*(-real(Xdcpnz_c(:,i+1))'*T213*real(Ydcpnz_c(:,j+1)) + imag(Xdcpnz_c(:,i+1))'*T213*imag(Ydcpnz_c(:,j+1)) ...
                                                           - real(Xdcpnz_c(:,j+1))'*T213*real(Ydcpnz_c(:,i+1)) + imag(Xdcpnz_c(:,j+1))'*T213*imag(Ydcpnz_c(:,i+1)));

                    Zdcpnz_c(1,h+1) = Zdcpnz_c(1,h+1) + 0.5*(real(Xdcpnz_c([1,3],i+1))'*[0 1; 1 0]*imag(Ydcpnz_c([1,3],j+1)) + imag(Xdcpnz_c([1,3],i+1))'*[0 1; 1 0]*real(Ydcpnz_c([1,3],j+1)) ...
                                                           + real(Xdcpnz_c([1,3],j+1))'*[0 1; 1 0]*imag(Ydcpnz_c([1,3],i+1)) + imag(Xdcpnz_c([1,3],j+1))'*[0 1; 1 0]*real(Ydcpnz_c([1,3],i+1)) );

                    Zdcpnz_c(1,h+1) = Zdcpnz_c(1,h+1) + 1i*0.5*(-real(Xdcpnz_c([1,3],i+1))'*[0 1; 1 0]*real(Ydcpnz_c([1,3],j+1)) + imag(Xdcpnz_c([1,3],i+1))'*[0 1; 1 0]*imag(Ydcpnz_c([1,3],j+1)) ...
                                                              - real(Xdcpnz_c([1,3],j+1))'*[0 1; 1 0]*real(Ydcpnz_c([1,3],i+1)) + imag(Xdcpnz_c([1,3],j+1))'*[0 1; 1 0]*imag(Ydcpnz_c([1,3],i+1)) );

                    Zdcpnz_c(2,h+1) = Zdcpnz_c(2,h+1) + 0.5*(real(Xdcpnz_c([2,3],i+1))'*[0 1; 1 0]*imag(Ydcpnz_c([2,3],j+1)) + imag(Xdcpnz_c([2,3],i+1))'*[0 1; 1 0]*real(Ydcpnz_c([2,3],j+1)) ...
                                                           + real(Xdcpnz_c([2,3],j+1))'*[0 1; 1 0]*imag(Ydcpnz_c([2,3],i+1)) + imag(Xdcpnz_c([2,3],j+1))'*[0 1; 1 0]*real(Ydcpnz_c([2,3],i+1)) );

                    Zdcpnz_c(2,h+1) = Zdcpnz_c(2,h+1) + 1i*0.5*(-real(Xdcpnz_c([2,3],i+1))'*[0 1; 1 0]*real(Ydcpnz_c([2,3],j+1)) + imag(Xdcpnz_c([2,3],i+1))'*[0 1; 1 0]*imag(Ydcpnz_c([2,3],j+1)) ...
                                                              - real(Xdcpnz_c([2,3],j+1))'*[0 1; 1 0]*real(Ydcpnz_c([2,3],i+1)) + imag(Xdcpnz_c([2,3],j+1))'*[0 1; 1 0]*imag(Ydcpnz_c([2,3],i+1)) );

                end
%%%%%%%%%%%%%%%%%%%%%% h<=N EVEN %%%%%%%%%%%%%%%%%%%%%%%%%%%%%%%%%%%%%%%%%           
            else  

                Zdcpnz_c(3,h+1) = Zdcpnz_c(3,h+1) + 0.5*imag(Xdcpnz_c(3,h/2+1)*Ydcpnz_c(3,h/2+1))           -0.5*1i*real(Xdcpnz_c(3,h/2+1)*Ydcpnz_c(3,h/2+1));
                Zdcpnz_c(1,h+1) = Zdcpnz_c(1,h+1) + 0.5*real(Xdcpnz_c(:,h/2+1))'*T321*imag(Ydcpnz_c(:,h/2+1)) + 0.5*imag(Xdcpnz_c(:,h/2+1))'*T321*real(Ydcpnz_c(:,h/2+1));
                Zdcpnz_c(1,h+1) = Zdcpnz_c(1,h+1) - 0.5*1i*real(Xdcpnz_c(:,h/2+1))'*T321*real(Ydcpnz_c(:,h/2+1)) + 0.5*1i*imag(Xdcpnz_c(:,h/2+1))'*T321*imag(Ydcpnz_c(:,h/2+1));
                Zdcpnz_c(2,h+1) = Zdcpnz_c(2,h+1) + 0.5*real(Xdcpnz_c(:,h/2+1))'*T132*imag(Ydcpnz_c(:,h/2+1)) + 0.5*imag(Xdcpnz_c(:,h/2+1))'*T132*real(Ydcpnz_c(:,h/2+1));
                Zdcpnz_c(2,h+1) = Zdcpnz_c(2,h+1) - 0.5*1i*real(Xdcpnz_c(:,h/2+1))'*T132*real(Ydcpnz_c(:,h/2+1)) + 0.5*1i*imag(Xdcpnz_c(:,h/2+1))'*T132*imag(Ydcpnz_c(:,h/2+1));
                
                for k = 1:N-h
                    i = k;
                    j = h+i;

                    Zdcpnz_c(1,h+1) = Zdcpnz_c(1,h+1) + 0.5*( - real(Xdcpnz_c(:,i+1))'*T231*imag(Ydcpnz_c(:,j+1)) + imag(Xdcpnz_c(:,i+1))'*T231*real(Ydcpnz_c(:,j+1)) ...
                                                              + real(Xdcpnz_c(:,j+1))'*T312*imag(Ydcpnz_c(:,i+1)) - imag(Xdcpnz_c(:,j+1))'*T312*real(Ydcpnz_c(:,i+1)));

                    Zdcpnz_c(1,h+1) = Zdcpnz_c(1,h+1) + 0.5*1i*( + real(Xdcpnz_c(:,i+1))'*T231*real(Ydcpnz_c(:,j+1)) + imag(Xdcpnz_c(:,i+1))'*T231*imag(Ydcpnz_c(:,j+1)) ...
                                                                 + real(Xdcpnz_c(:,j+1))'*T312*real(Ydcpnz_c(:,i+1)) + imag(Xdcpnz_c(:,j+1))'*T312*imag(Ydcpnz_c(:,i+1)));

                    Zdcpnz_c(2,h+1) = Zdcpnz_c(2,h+1) + 0.5*( - real(Xdcpnz_c(:,i+1))'*T312*imag(Ydcpnz_c(:,j+1)) + imag(Xdcpnz_c(:,i+1))'*T312*real(Ydcpnz_c(:,j+1)) ...
                                                              + real(Xdcpnz_c(:,j+1))'*T231*imag(Ydcpnz_c(:,i+1)) - imag(Xdcpnz_c(:,j+1))'*T231*real(Ydcpnz_c(:,i+1)));

                    Zdcpnz_c(2,h+1) = Zdcpnz_c(2,h+1) + 1i*0.5*( + real(Xdcpnz_c(:,i+1))'*T312*real(Ydcpnz_c(:,j+1)) + imag(Xdcpnz_c(:,i+1))'*T312*imag(Ydcpnz_c(:,j+1)) ...
                                                              + real(Xdcpnz_c(:,j+1))'*T231*real(Ydcpnz_c(:,i+1)) + imag(Xdcpnz_c(:,j+1))'*T231*imag(Ydcpnz_c(:,i+1)));

                    Zdcpnz_c(3,h+1) = Zdcpnz_c(3,h+1) + 0.5*(-real(Xdcpnz_c(:,i+1))'*imag(Ydcpnz_c(:,j+1))+imag(Xdcpnz_c(:,i+1))'*real(Ydcpnz_c(:,j+1)) ...
                                                             +real(Xdcpnz_c(:,j+1))'*imag(Ydcpnz_c(:,i+1))-imag(Xdcpnz_c(:,j+1))'*real(Ydcpnz_c(:,i+1)));

                    Zdcpnz_c(3,h+1) = Zdcpnz_c(3,h+1) + 0.5*1i*(+real(Xdcpnz_c(:,i+1))'*real(Ydcpnz_c(:,j+1))+imag(Xdcpnz_c(:,i+1))'*imag(Ydcpnz_c(:,j+1)) ...
                                                             +real(Xdcpnz_c(:,j+1))'*real(Ydcpnz_c(:,i+1))+imag(Xdcpnz_c(:,j+1))'*imag(Ydcpnz_c(:,i+1)));

                end

                for k = h/2-1:-1:1
                    i = k;
                    j = h-i;   

                    Zdcpnz_c(3,h+1) = Zdcpnz_c(3,h+1) +    0.5*(+real(Xdcpnz_c(:,i+1))'*T213*imag(Ydcpnz_c(:,j+1)) + real(Xdcpnz_c(:,j+1))'*T213*imag(Ydcpnz_c(:,i+1)) + imag(Xdcpnz_c(:,i+1))'*T213*real(Ydcpnz_c(:,j+1)) + imag(Xdcpnz_c(:,j+1))'*T213*real(Ydcpnz_c(:,i+1)));

                    Zdcpnz_c(3,h+1) = Zdcpnz_c(3,h+1) + 1i*0.5*(-real(Xdcpnz_c(:,i+1))'*T213*real(Ydcpnz_c(:,j+1)) - real(Xdcpnz_c(:,j+1))'*T213*real(Ydcpnz_c(:,i+1)) + imag(Xdcpnz_c(:,i+1))'*T213*imag(Ydcpnz_c(:,j+1)) + imag(Xdcpnz_c(:,j+1))'*T213*imag(Ydcpnz_c(:,i+1)));

                    Zdcpnz_c(1,h+1) = Zdcpnz_c(1,h+1) + 0.5*( + real(Xdcpnz_c(:,i+1))'*T321*imag(Ydcpnz_c(:,j+1)) + imag(Xdcpnz_c(:,i+1))'*T321*real(Ydcpnz_c(:,j+1)) ...
                                                              + real(Xdcpnz_c(:,j+1))'*T321*imag(Ydcpnz_c(:,i+1)) + imag(Xdcpnz_c(:,j+1))'*T321*real(Ydcpnz_c(:,i+1)));


                    Zdcpnz_c(1,h+1) = Zdcpnz_c(1,h+1) + 0.5*1i*( - real(Xdcpnz_c(:,i+1))'*T321*real(Ydcpnz_c(:,j+1)) + imag(Xdcpnz_c(:,i+1))'*T321*imag(Ydcpnz_c(:,j+1)) ...
                                                                 - real(Xdcpnz_c(:,j+1))'*T321*real(Ydcpnz_c(:,i+1)) + imag(Xdcpnz_c(:,j+1))'*T321*imag(Ydcpnz_c(:,i+1)));
                    
                    Zdcpnz_c(2,h+1) = Zdcpnz_c(2,h+1) + 0.5*( + real(Xdcpnz_c(:,i+1))'*T132*imag(Ydcpnz_c(:,j+1)) + imag(Xdcpnz_c(:,i+1))'*T132*real(Ydcpnz_c(:,j+1)) ...
                                                              + real(Xdcpnz_c(:,j+1))'*T132*imag(Ydcpnz_c(:,i+1)) + imag(Xdcpnz_c(:,j+1))'*T132*real(Ydcpnz_c(:,i+1)));

                    Zdcpnz_c(2,h+1) = Zdcpnz_c(2,h+1) + 1i*0.5*( - real(Xdcpnz_c(:,i+1))'*T132*real(Ydcpnz_c(:,j+1)) + imag(Xdcpnz_c(:,i+1))'*T132*imag(Ydcpnz_c(:,j+1)) ...
                                                                 - real(Xdcpnz_c(:,j+1))'*T132*real(Ydcpnz_c(:,i+1)) + imag(Xdcpnz_c(:,j+1))'*T132*imag(Ydcpnz_c(:,i+1)));

                end
            end
%%%%%%%%%%%%%%%%%%%%%%%%%%%% h>N  %%%%%%%%%%%%%%%%%%%%%%%%%%%%%%%%%%%%%%%%% 
        else %h>N
            if(HrmDbl)
            
                %%%%%%%%%%%%%%%%%%%%%%%%%%% PP + NN %%%%%%%%%%%%%%%%%%%%%%%%%%%
                for i = h-N : N
                    Zdcpnz_c(1,h+1) = Zdcpnz_c(1,h+1) +    0.5*( real(Xdcpnz_c(2,i+1))*imag(Ydcpnz_c(2,h-i+1)) + imag(Xdcpnz_c(2,i+1))*real(Ydcpnz_c(2,h-i+1)) );
                    Zdcpnz_c(1,h+1) = Zdcpnz_c(1,h+1) + 1i*0.5*( -real(Xdcpnz_c(2,i+1))*real(Ydcpnz_c(2,h-i+1)) + imag(Xdcpnz_c(2,i+1))*imag(Ydcpnz_c(2,h-i+1)) );

                    Zdcpnz_c(2,h+1) = Zdcpnz_c(2,h+1) +    0.5*( real(Xdcpnz_c(1,i+1))*imag(Ydcpnz_c(1,h-i+1)) + imag(Xdcpnz_c(1,i+1))*real(Ydcpnz_c(1,h-i+1)) );
                    Zdcpnz_c(2,h+1) = Zdcpnz_c(2,h+1) + 1i*0.5*( -real(Xdcpnz_c(1,i+1))*real(Ydcpnz_c(1,h-i+1)) + imag(Xdcpnz_c(1,i+1))*imag(Ydcpnz_c(1,h-i+1)) );
                end
                %%%%%%%%%%%%%%%%%%%%%%%%%%% PP + NN %%%%%%%%%%%%%%%%%%%%%%%%%%%

                if(mod(h,2)==1) %%%%%%%%%%% h>N ODD %%%%%%%%%%%%%%%%%%%

                    for k = (h-1)/2:-1:h-N
                        i = k;  %%%
                        j = h-i;

                        Zdcpnz_c(1,h+1) = Zdcpnz_c(1,h+1) + 0.5*( + real(Xdcpnz_c([1,3],i+1))'*imag(Ydcpnz_c([3,1],j+1)) + imag(Xdcpnz_c([1,3],i+1))'*real(Ydcpnz_c([3,1],j+1)) ...
                                                                  + real(Xdcpnz_c([1,3],j+1))'*imag(Ydcpnz_c([3,1],i+1)) + imag(Xdcpnz_c([1,3],j+1))'*real(Ydcpnz_c([3,1],i+1)));

                        Zdcpnz_c(1,h+1) = Zdcpnz_c(1,h+1) + 1i*0.5*( - real(Xdcpnz_c([1,3],i+1))'*real(Ydcpnz_c([3,1],j+1)) + imag(Xdcpnz_c([1,3],i+1))'*imag(Ydcpnz_c([3,1],j+1)) ...
                                                                     - real(Xdcpnz_c([1,3],j+1))'*real(Ydcpnz_c([3,1],i+1)) + imag(Xdcpnz_c([1,3],j+1))'*imag(Ydcpnz_c([3,1],i+1)));

                        Zdcpnz_c(2,h+1) = Zdcpnz_c(2,h+1) + 0.5*( + real(Xdcpnz_c([2,3],i+1))'*imag(Ydcpnz_c([3,2],j+1)) + imag(Xdcpnz_c([2,3],i+1))'*real(Ydcpnz_c([3,2],j+1)) ...
                                                                  + real(Xdcpnz_c([2,3],j+1))'*imag(Ydcpnz_c([3,2],i+1)) + imag(Xdcpnz_c([2,3],j+1))'*real(Ydcpnz_c([3,2],i+1)));

                        Zdcpnz_c(2,h+1) = Zdcpnz_c(2,h+1) + 1i*0.5*( - real(Xdcpnz_c([2,3],i+1))'*real(Ydcpnz_c([3,2],j+1)) + imag(Xdcpnz_c([2,3],i+1))'*imag(Ydcpnz_c([3,2],j+1)) ...
                                                                     - real(Xdcpnz_c([2,3],j+1))'*real(Ydcpnz_c([3,2],i+1)) + imag(Xdcpnz_c([2,3],j+1))'*imag(Ydcpnz_c([3,2],i+1)));

                        Zdcpnz_c(3,h+1) = Zdcpnz_c(3,h+1) +    0.5*(+real(Xdcpnz_c(:,i+1))'*T213*imag(Ydcpnz_c(:,j+1)) + real(Xdcpnz_c(:,j+1))'*T213*imag(Ydcpnz_c(:,i+1)) + imag(Xdcpnz_c(:,i+1))'*T213*real(Ydcpnz_c(:,j+1)) + imag(Xdcpnz_c(:,j+1))'*T213*real(Ydcpnz_c(:,i+1)));
                        Zdcpnz_c(3,h+1) = Zdcpnz_c(3,h+1) + 1i*0.5*(-real(Xdcpnz_c(:,i+1))'*T213*real(Ydcpnz_c(:,j+1)) - real(Xdcpnz_c(:,j+1))'*T213*real(Ydcpnz_c(:,i+1)) + imag(Xdcpnz_c(:,i+1))'*T213*imag(Ydcpnz_c(:,j+1)) + imag(Xdcpnz_c(:,j+1))'*T213*imag(Ydcpnz_c(:,i+1)));

                    end

                else %%%%%%%%%%% h>N EVEN %%%%%%%%%%%%%%%%%%%

                    Zdcpnz_c(1,h+1) = 0.5*real(Xdcpnz_c(:,h/2+1))'*T321*imag(Ydcpnz_c(:,h/2+1)) + 0.5*imag(Xdcpnz_c(:,h/2+1))'*T321*real(Ydcpnz_c(:,h/2+1)) - 0.5*1i*real(Xdcpnz_c(:,h/2+1))'*T321*real(Ydcpnz_c(:,h/2+1)) + 0.5*1i*imag(Xdcpnz_c(:,h/2+1))'*T321*imag(Ydcpnz_c(:,h/2+1));
                    Zdcpnz_c(2,h+1) = 0.5*real(Xdcpnz_c(:,h/2+1))'*T132*imag(Ydcpnz_c(:,h/2+1)) + 0.5*imag(Xdcpnz_c(:,h/2+1))'*T132*real(Ydcpnz_c(:,h/2+1))- 0.5*1i*real(Xdcpnz_c(:,h/2+1))'*T132*real(Ydcpnz_c(:,h/2+1)) + 0.5*1i*imag(Xdcpnz_c(:,h/2+1))'*T132*imag(Ydcpnz_c(:,h/2+1));
                    Zdcpnz_c(3,h+1) = Zdcpnz_c(3,h+1) + 0.5*imag(Xdcpnz_c(3,h/2+1)*Ydcpnz_c(3,h/2+1)) - 1i*0.5*real(Xdcpnz_c(3,h/2+1)*Ydcpnz_c(3,h/2+1));


                    for i = (h+2)/2:N
                        j = h-i;

                        Zdcpnz_c(1,h+1) = Zdcpnz_c(1,h+1) + 0.5*( + real(Xdcpnz_c(:,i+1))'*T321*imag(Ydcpnz_c(:,j+1)) + imag(Xdcpnz_c(:,i+1))'*T321*real(Ydcpnz_c(:,j+1)) ...
                                                                  + real(Xdcpnz_c(:,j+1))'*T321*imag(Ydcpnz_c(:,i+1)) + imag(Xdcpnz_c(:,j+1))'*T321*real(Ydcpnz_c(:,i+1)));
    
                        Zdcpnz_c(1,h+1) = Zdcpnz_c(1,h+1) + 0.5*1i*( - real(Xdcpnz_c(:,i+1))'*T321*real(Ydcpnz_c(:,j+1)) + imag(Xdcpnz_c(:,i+1))'*T321*imag(Ydcpnz_c(:,j+1)) ...
                                                                     - real(Xdcpnz_c(:,j+1))'*T321*real(Ydcpnz_c(:,i+1)) + imag(Xdcpnz_c(:,j+1))'*T321*imag(Ydcpnz_c(:,i+1)));

                        Zdcpnz_c(2,h+1) = Zdcpnz_c(2,h+1) + 0.5*( + real(Xdcpnz_c(:,i+1))'*T132*imag(Ydcpnz_c(:,j+1)) + imag(Xdcpnz_c(:,i+1))'*T132*real(Ydcpnz_c(:,j+1)) ...
                                                                  + real(Xdcpnz_c(:,j+1))'*T132*imag(Ydcpnz_c(:,i+1)) + imag(Xdcpnz_c(:,j+1))'*T132*real(Ydcpnz_c(:,i+1)));
    
                        Zdcpnz_c(2,h+1) = Zdcpnz_c(2,h+1) + 0.5*1i*( - real(Xdcpnz_c(:,i+1))'*T132*real(Ydcpnz_c(:,j+1)) + imag(Xdcpnz_c(:,i+1))'*T132*imag(Ydcpnz_c(:,j+1)) ...
                                                                     - real(Xdcpnz_c(:,j+1))'*T132*real(Ydcpnz_c(:,i+1)) + imag(Xdcpnz_c(:,j+1))'*T132*imag(Ydcpnz_c(:,i+1)));

                        Zdcpnz_c(3,h+1) = Zdcpnz_c(3,h+1) +    0.5*(+real(Xdcpnz_c(:,i+1))'*T213*imag(Ydcpnz_c(:,j+1)) + real(Xdcpnz_c(:,j+1))'*T213*imag(Ydcpnz_c(:,i+1)) + imag(Xdcpnz_c(:,i+1))'*T213*real(Ydcpnz_c(:,j+1)) + imag(Xdcpnz_c(:,j+1))'*T213*real(Ydcpnz_c(:,i+1)));
                        Zdcpnz_c(3,h+1) = Zdcpnz_c(3,h+1) + 1i*0.5*(-real(Xdcpnz_c(:,i+1))'*T213*real(Ydcpnz_c(:,j+1)) - real(Xdcpnz_c(:,j+1))'*T213*real(Ydcpnz_c(:,i+1)) + imag(Xdcpnz_c(:,i+1))'*T213*imag(Ydcpnz_c(:,j+1)) + imag(Xdcpnz_c(:,j+1))'*T213*imag(Ydcpnz_c(:,i+1)));

                    end
                end
            end
        end  
    end
    

end

== matlab function P2PHVDCMMC/DQn->ABC1 ==
  settings: updateMethod=DISCRETE
  data: Xdcpnz_c input; tho input; Xabc output; N parameter
%function abc = Mult(Z0,Zdp,Zqp,Zdn,Zqn,Zdz,Zqz,th, N)
function Xabc = dqn2abc(Xdcpnz_c,tho,N)

    persistent Sas;
    persistent Ssa;

    if(isempty(Sas)) 
        a = -0.5+0.866i;
        a2 = -0.5-0.866i;
        Sas = [1,a,a2;1,a2,a;1,1,1]/3;
        Ssa = eye(3)/(Sas);
    end

    Xabc = zeros(3,1);

    for i = 1 : N+1
    
    
        if(i>1)
            h = i-1;
    
            th = h*tho;
        
            mag_p = abs(Xdcpnz_c(1,i));
            ang_p = angle(Xdcpnz_c(1,i));
            mag_n = abs(Xdcpnz_c(2,i));
            ang_n = angle(Xdcpnz_c(2,i));
            mag_z = abs(Xdcpnz_c(3,i));
            ang_z = angle(Xdcpnz_c(3,i));
            
            abc3p = mag_p*[sin(th+ang_p) ; sin(th+ang_p-2*pi/3) ; sin(th+ang_p+2*pi/3) ];
            abc3n = mag_n*[sin(th+ang_n) ; sin(th+ang_n+2*pi/3) ; sin(th+ang_n-2*pi/3) ];
            abc3z = mag_z*[sin(th+ang_z) ; sin(th+ang_z)        ; sin(th+ang_z)  ];
        
            Xabc = Xabc + abc3p+abc3n+abc3z;
        else
            Xabc = Xabc + real(Ssa*(Xdcpnz_c(:,1)));
        
        end
    
        
    end

end

== matlab function P2PHVDCMMC/Subsystem4/ACrec/Int_DQNc_Mat1 ==
  settings: updateMethod=DISCRETE
  data: Xpnz input; N parameter; dt parameter; w parameter; InitInt parameter; Zpnz output; R parameter; iL parameter; swFeed parameter
function Zpnz    = Int_DQN_Mat(Xpnz, N, dt, w, InitInt, R, iL, swFeed)


    nrSig = size(Xpnz,1)/3;
    Zpnz = complex(zeros(nrSig*3,N+1));

    persistent Zpnz_old;
    persistent Xpnz_old;
    persistent Krl1;
    persistent Krl2;
    persistent dt2;
        
    if(isempty(Zpnz_old)) 
    


        
        % if(~isempty(InitInt))
        % Zpnz_old(:,1) = Sas * InitInt;
        % end


        Zpnz_old = complex(zeros(nrSig*3,N+1));
        Xpnz_old = complex(zeros(nrSig*3,N+1));
        dt2 = dt/2;

        if(swFeed)
            mrows = size(R,1)/3; %signal size
            mcols = size(R,2)/3; %signal size

            szMatR = size(R,1);
            szMatiL = size(iL,1);

            if(szMatiL ~= szMatR || size(R,1) ~= size(R,2) || size(iL,1) ~= size(iL,2))
                error('[Int_DQN_Mat/swFeedback] check matrix sizes!');
            end
    
            Rpnz = complex(zeros(3*mrows,3*mcols));
            iLpnz = complex(zeros(3*mrows,3*mcols));

            a = -0.5+0.866i;
            a2 = -0.5-0.866i;
            Sas = [1,a,a2;1,a2,a;1,1,1]/3;
    
            for i = 1 : mrows
                for j = 1 : mcols
                     Rpnz((1:3) + (i-1)*3,(1:3) + (j-1)*3) = Sas*R((1:3) + (i-1)*3,(1:3) + (j-1)*3)/Sas;
                    iLpnz((1:3) + (i-1)*3,(1:3) + (j-1)*3) = Sas*iL((1:3) + (i-1)*3,(1:3) + (j-1)*3)/Sas;
                end
            end

            Rpnz  = diag(diag(real(Rpnz)));
            iLpnz = diag(diag(real(iLpnz)));

            Krl1 = (iLpnz/(eye(szMatR)+dt2*Rpnz*iLpnz));
            Krl2 = (eye(szMatR)-dt2*Rpnz*iLpnz)/(eye(szMatR)+dt2*Rpnz*iLpnz);
        else
            Krl1 = 1;
            Krl2 = 1;
        end
            
    end

    if(swFeed)
        Zpnz(:,1) = Krl1*dt2*(Xpnz(:,1)+Xpnz_old(:,1))+Krl2*Zpnz_old(:,1);
    else
        Zpnz(:,1) = dt2*(Xpnz(:,1)+Xpnz_old(:,1))+Zpnz_old(:,1);
    end

    Xpnz_old(:,1) = Xpnz(:,1);
    Zpnz_old(:,1) = Zpnz(:,1);

    for i = 1 : N
        if(N>0)
            wn =  i * w; 
            wndt2 = wn*dt2;

            A = 2*dt2/(1+wndt2^2);
            B = (1-wndt2^2)/(1+wndt2^2);

            if(swFeed)

                Zpnz(:,i+1) =      Krl1*A*(real(Xpnz(:,i+1))+wndt2*imag(Xpnz(:,i+1)))+Krl2*(B*real(Zpnz_old(:,i+1))+A*wn*imag(Zpnz_old(:,i+1))) ...
                             + 1i*(Krl1*A*(imag(Xpnz(:,i+1))-wndt2*real(Xpnz(:,i+1)))+Krl2*(B*imag(Zpnz_old(:,i+1))-A*wn*real(Zpnz_old(:,i+1))));
            else
                Zpnz(:,i+1) =      A*(real(Xpnz(:,i+1))+wndt2*imag(Xpnz(:,i+1)))+(B*real(Zpnz_old(:,i+1))+A*wn*imag(Zpnz_old(:,i+1))) ...
                             + 1i*(A*(imag(Xpnz(:,i+1))-wndt2*real(Xpnz(:,i+1)))+(B*imag(Zpnz_old(:,i+1))-A*wn*real(Zpnz_old(:,i+1))));
            end

            Zpnz_old(:,i+1) = Zpnz(:,i+1);

        end
    end


end
